simulink model "cdmatest3"  (R2020a)
settings: Solver=VariableStepAuto  StartTime=0.0  StopTime=10  RelTol=1e-3
libraries: commutil2 x20, commdigbbndpm3 x8, commrandsrc3 x8, commseqgen3 x8, commsink2 x4, dsparch4 x4, commchan3 x1
settings Model: Creator=xxy15334437753  LastModifiedBy=xxy15334437753

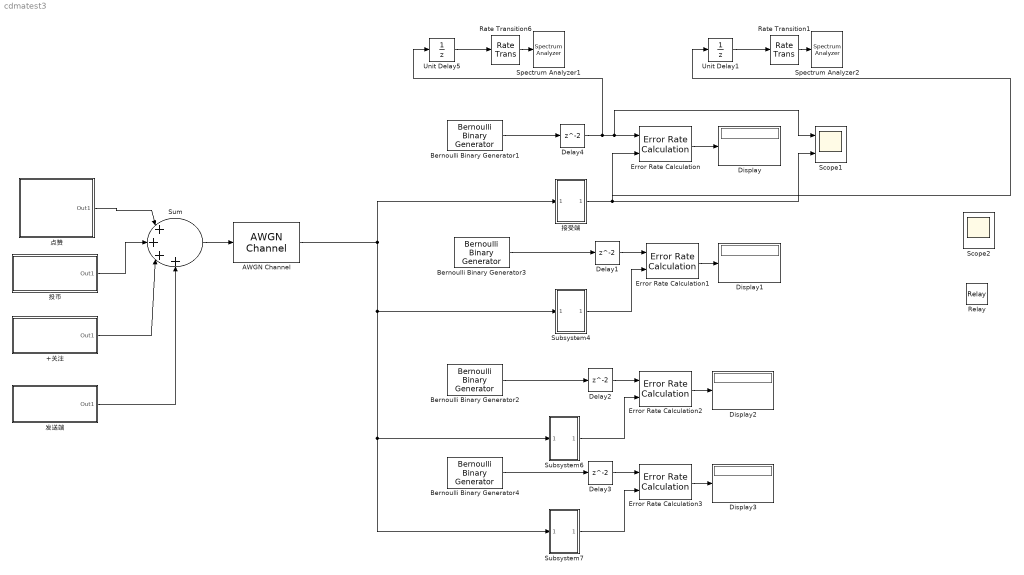
== system cdmatest3 ==
  +关注 : Subsystem
  AWGN Channel : commchan3/AWGN Channel  InputProcessing=Columns as channels (frame based)  seed=67  noiseMode="Signal to noise ratio  (Eb/No)"  EbNodB=10  EsNodB=10  SNRdB=20  bitsPerSym=1  Ps=1  Tsym=1/6400  variance=5
  Bernoulli Binary Generator1 : commrandsrc3/Bernoulli Binary Generator  ProbabilityOfZero=0.5  SeedSource=Parameter  Seed=88  SampleTime=0.01  SamplesPerFrame=1  OutputDataType=double  SimulateUsing=Code generation
  Bernoulli Binary Generator2 : commrandsrc3/Bernoulli Binary Generator  ProbabilityOfZero=0.5  SeedSource=Parameter  Seed=110  SampleTime=0.01  SamplesPerFrame=1  OutputDataType=double  SimulateUsing=Code generation
  Bernoulli Binary Generator3 : commrandsrc3/Bernoulli Binary Generator  ProbabilityOfZero=0.5  SeedSource=Parameter  Seed=67  SampleTime=0.01  SamplesPerFrame=1  OutputDataType=double  SimulateUsing=Code generation
  Bernoulli Binary Generator4 : commrandsrc3/Bernoulli Binary Generator  ProbabilityOfZero=0.5  SeedSource=Parameter  Seed=120  SampleTime=0.01  SamplesPerFrame=1  OutputDataType=double  SimulateUsing=Code generation
  Delay{1..4} (4 alike) : Delay
  Display{,1..3} (4 alike) : Display
  Error Rate Calculation{,1..3} (4 alike) : commsink2/Error Rate Calculation  N=0  st_delay=0  cp_mode=Entire frame  subframe=[]  PMode=Port  WsName=ErrorVec  RsMode2=off  stop=off  numErr=100  maxBits=1e6
  Rate Transition1 : RateTransition  OutPortSampleTime=1/3200
  Rate Transition6 : RateTransition  OutPortSampleTime=1/3200
  Relay : Relay
  Scope1 : Scope  NumInputPorts=2
  Scope2 : Scope  NumInputPorts=2
  Spectrum Analyzer1 : SpectrumAnalyzer
  Spectrum Analyzer2 : SpectrumAnalyzer
  Subsystem4 : Subsystem
  Subsystem6 : Subsystem
  Subsystem7 : Subsystem
  Sum : Sum  Inputs=|++++  OutMin=[-1]  OutMax=[1]  OutDataTypeStr=double
  Unit Delay1 : UnitDelay  SampleTime=-1  HasFrameUpgradeWarning=on
  Unit Delay5 : UnitDelay  SampleTime=-1  HasFrameUpgradeWarning=on
  发送端 : Subsystem
  投币 : Subsystem
  接受端 : Subsystem
  点赞 : Subsystem
  wires:
  Error Rate Calculation/1 -> Display/1
  Error Rate Calculation1/1 -> Display1/1
  Sum/1 -> AWGN Channel/1
  点赞/1(Out1) -> Sum/1
  投币/1(Out1) -> Sum/2
  +关注/1(Out1) -> Sum/3
  Bernoulli Binary Generator1/1 -> Delay4/1
  Bernoulli Binary Generator3/1 -> Delay1/1
  Delay1/1 -> Error Rate Calculation1/1
  Subsystem4/1(Out1) -> Error Rate Calculation1/2
  Subsystem6/1(Out1) -> Error Rate Calculation2/2
  Delay2/1 -> Error Rate Calculation2/1
  Bernoulli Binary Generator2/1 -> Delay2/1
  Error Rate Calculation2/1 -> Display2/1
  Error Rate Calculation3/1 -> Display3/1
  Bernoulli Binary Generator4/1 -> Delay3/1
  Delay3/1 -> Error Rate Calculation3/1
  Subsystem7/1(Out1) -> Error Rate Calculation3/2
  AWGN Channel/1 -> Subsystem7/1(In1), Subsystem6/1(In1), Subsystem4/1(In1), 接受端/1(In1)
  发送端/1(Out1) -> Sum/4
  Rate Transition6/1 -> Spectrum Analyzer1/1
  Delay4/1 -> Unit Delay5/1, Scope1/1, Error Rate Calculation/1
  Unit Delay5/1 -> Rate Transition6/1
  接受端/1(Out1) -> Unit Delay1/1, Scope1/2, Error Rate Calculation/2
  Rate Transition1/1 -> Spectrum Analyzer2/1
  Unit Delay1/1 -> Rate Transition1/1

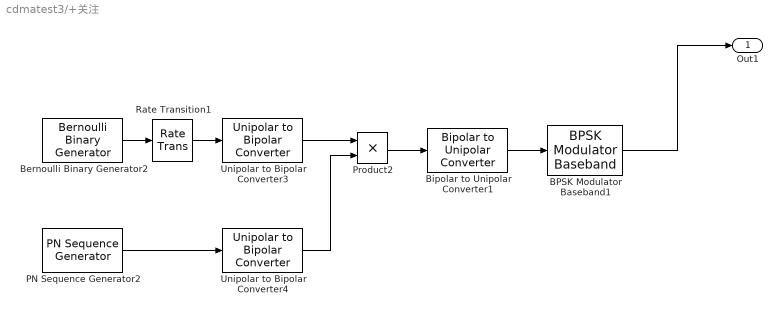
== system cdmatest3/+关注 ==
  BPSK Modulator Baseband1 : commdigbbndpm3/BPSK Modulator Baseband  Ph=0  outDtype=double  outWordLen=16  outUDDataType=sfix(16)  outFracLenMode=Best precision  outFracLen=15  outDataTypeStr=double  outLastDataTypeStr=double
  Bernoulli Binary Generator2 : commrandsrc3/Bernoulli Binary Generator  ProbabilityOfZero=0.5  SeedSource=Parameter  Seed=110  SampleTime=0.01  SamplesPerFrame=1  OutputDataType=double  SimulateUsing=Code generation
  Bipolar to Unipolar Converter1 : commutil2/Bipolar to Unipolar Converter  M=2  polarity=Positive  dataType=double
      settings: SourceProductBaseCode=CM
  PN Sequence Generator2 : commseqgen3/PN Sequence Generator  poly=[1 0 0 0 0 0 1 1]  ini_sta=[1 1 0 0 1 0 1]  outBitMaskSource=Dialog parameter  shift=0  outVarSiz=off  maxOutSizeMode=Dialog parameter  maxOutSize=[10 1]  Ts=1/6400  sampPerFrame=1  reset=off  bitPackedOutputs=off  outDataType=double  numPackedBits=8  bitPackDataSigned=off  bitPackedOutDType=double
  Product2 : Product
  Rate Transition1 : RateTransition  OutPortSampleTimeMultiple=20  OutPortSampleTime=1/3200
  Unipolar to Bipolar Converter3 : commutil2/Unipolar to Bipolar Converter  M=2  polarity=Positive  dataType=Inherit via internal rule
  Unipolar to Bipolar Converter4 : commutil2/Unipolar to Bipolar Converter  M=2  polarity=Positive  dataType=Inherit via internal rule
  Out1 : Outport
  wires:
  Rate Transition1/1 -> Unipolar to Bipolar Converter3/1
  BPSK Modulator Baseband1/1 -> Out1/1
  Bernoulli Binary Generator2/1 -> Rate Transition1/1
  Bipolar to Unipolar Converter1/1 -> BPSK Modulator Baseband1/1
  Unipolar to Bipolar Converter4/1 -> Product2/2
  Unipolar to Bipolar Converter3/1 -> Product2/1
  PN Sequence Generator2/1 -> Unipolar to Bipolar Converter4/1
  Product2/1 -> Bipolar to Unipolar Converter1/1

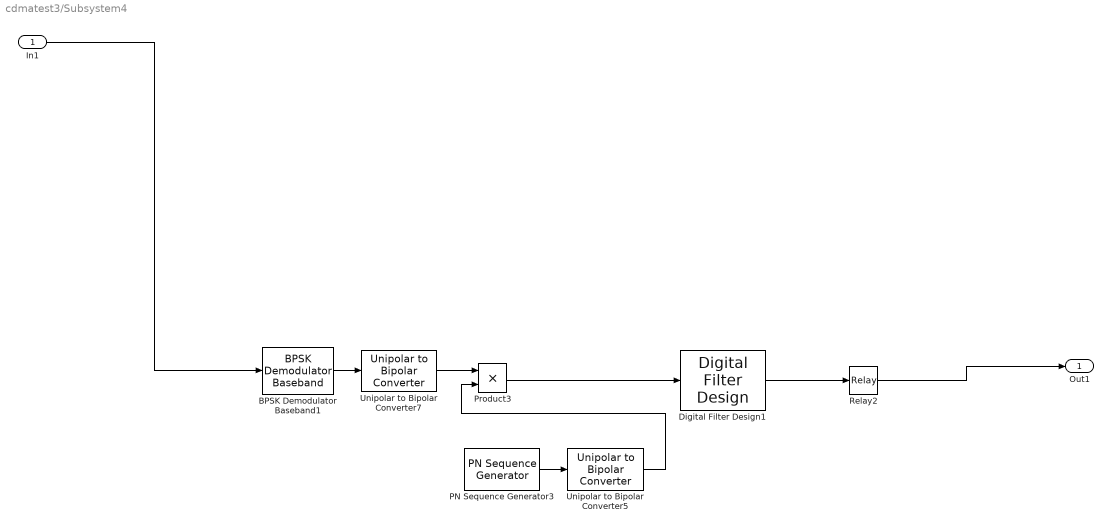
== system cdmatest3/Subsystem4 ==
  In1 : Inport
  BPSK Demodulator Baseband1 : commdigbbndpm3/BPSK Demodulator Baseband  DecType=Hard decision  VarSource=Dialog  Variance=1  Ph=0  outDtype=Inherit via internal rule  derotateFactorWordLen=16  derotateFactorDataTypeStr=Inherit: Same word length as input  derotateFactorLastDataTypeStr=Inherit: Same word length as input
  Digital Filter Design1 : dsparch4/Digital Filter Design  mwdsp_browser_bugfix_var=off
  PN Sequence Generator3 : commseqgen3/PN Sequence Generator  poly=[1 0 0 0 0 0 1 1]  ini_sta=[1 0 0 0 1 0 1]  outBitMaskSource=Dialog parameter  shift=0  outVarSiz=off  maxOutSizeMode=Dialog parameter  maxOutSize=[10 1]  Ts=1/6400  sampPerFrame=1  reset=off  bitPackedOutputs=off  outDataType=double  numPackedBits=8  bitPackDataSigned=off  bitPackedOutDType=double
  Product3 : Product
  Relay2 : Relay  OnSwitchValue=0  OffSwitchValue=0
  Unipolar to Bipolar Converter5 : commutil2/Unipolar to Bipolar Converter  M=2  polarity=Positive  dataType=Inherit via internal rule
  Unipolar to Bipolar Converter7 : commutil2/Unipolar to Bipolar Converter  M=2  polarity=Positive  dataType=Inherit via internal rule
  Out1 : Outport
  wires:
  PN Sequence Generator3/1 -> Unipolar to Bipolar Converter5/1
  In1/1 -> BPSK Demodulator Baseband1/1
  Product3/1 -> Digital Filter Design1/1
  Digital Filter Design1/1 -> Relay2/1
  Unipolar to Bipolar Converter5/1 -> Product3/2
  BPSK Demodulator Baseband1/1 -> Unipolar to Bipolar Converter7/1
  Unipolar to Bipolar Converter7/1 -> Product3/1
  Relay2/1 -> Out1/1

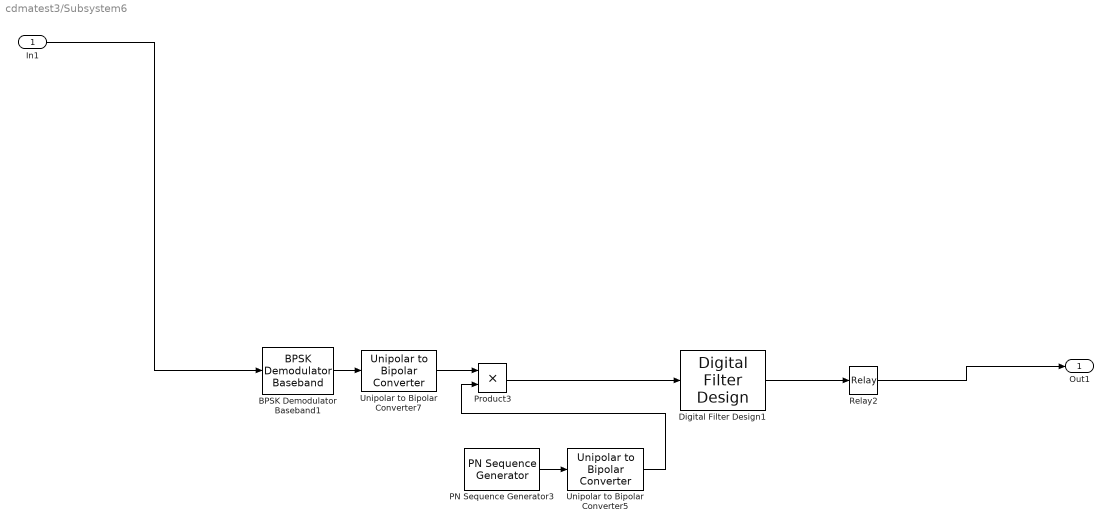
== system cdmatest3/Subsystem6 ==
  In1 : Inport
  BPSK Demodulator Baseband1 : commdigbbndpm3/BPSK Demodulator Baseband  DecType=Hard decision  VarSource=Dialog  Variance=1  Ph=0  outDtype=Inherit via internal rule  derotateFactorWordLen=16  derotateFactorDataTypeStr=Inherit: Same word length as input  derotateFactorLastDataTypeStr=Inherit: Same word length as input
  Digital Filter Design1 : dsparch4/Digital Filter Design  mwdsp_browser_bugfix_var=off
  PN Sequence Generator3 : commseqgen3/PN Sequence Generator  poly=[1 0 0 0 0 0 1 1]  ini_sta=[1 1 0 0 1 0 1]  outBitMaskSource=Dialog parameter  shift=0  outVarSiz=off  maxOutSizeMode=Dialog parameter  maxOutSize=[10 1]  Ts=1/6400  sampPerFrame=1  reset=off  bitPackedOutputs=off  outDataType=double  numPackedBits=8  bitPackDataSigned=off  bitPackedOutDType=double
  Product3 : Product
  Relay2 : Relay  OnSwitchValue=0  OffSwitchValue=0
  Unipolar to Bipolar Converter5 : commutil2/Unipolar to Bipolar Converter  M=2  polarity=Positive  dataType=Inherit via internal rule
  Unipolar to Bipolar Converter7 : commutil2/Unipolar to Bipolar Converter  M=2  polarity=Positive  dataType=Inherit via internal rule
  Out1 : Outport
  wires:
  Relay2/1 -> Out1/1
  Unipolar to Bipolar Converter7/1 -> Product3/1
  BPSK Demodulator Baseband1/1 -> Unipolar to Bipolar Converter7/1
  Unipolar to Bipolar Converter5/1 -> Product3/2
  Digital Filter Design1/1 -> Relay2/1
  Product3/1 -> Digital Filter Design1/1
  In1/1 -> BPSK Demodulator Baseband1/1
  PN Sequence Generator3/1 -> Unipolar to Bipolar Converter5/1

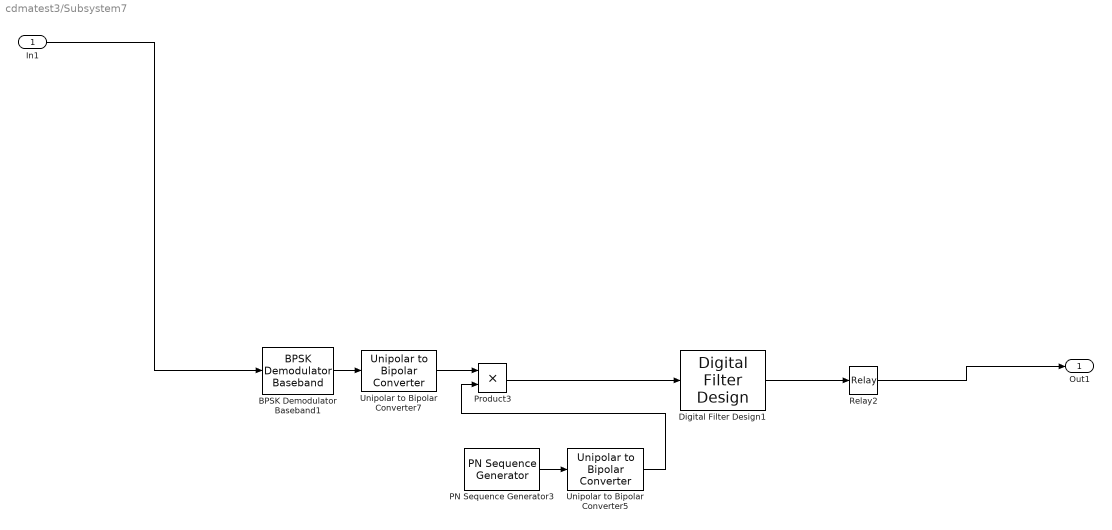
== system cdmatest3/Subsystem7 ==
  In1 : Inport
  BPSK Demodulator Baseband1 : commdigbbndpm3/BPSK Demodulator Baseband  DecType=Hard decision  VarSource=Dialog  Variance=1  Ph=0  outDtype=Inherit via internal rule  derotateFactorWordLen=16  derotateFactorDataTypeStr=Inherit: Same word length as input  derotateFactorLastDataTypeStr=Inherit: Same word length as input
  Digital Filter Design1 : dsparch4/Digital Filter Design  mwdsp_browser_bugfix_var=off
  PN Sequence Generator3 : commseqgen3/PN Sequence Generator  poly=[1 0 0 0 0 0 1 1]  ini_sta=[1 1 0 0 1 1 1]  outBitMaskSource=Dialog parameter  shift=0  outVarSiz=off  maxOutSizeMode=Dialog parameter  maxOutSize=[10 1]  Ts=1/6400  sampPerFrame=1  reset=off  bitPackedOutputs=off  outDataType=double  numPackedBits=8  bitPackDataSigned=off  bitPackedOutDType=double
  Product3 : Product
  Relay2 : Relay  OnSwitchValue=0  OffSwitchValue=0
  Unipolar to Bipolar Converter5 : commutil2/Unipolar to Bipolar Converter  M=2  polarity=Positive  dataType=Inherit via internal rule
  Unipolar to Bipolar Converter7 : commutil2/Unipolar to Bipolar Converter  M=2  polarity=Positive  dataType=Inherit via internal rule
  Out1 : Outport
  wires:
  PN Sequence Generator3/1 -> Unipolar to Bipolar Converter5/1
  In1/1 -> BPSK Demodulator Baseband1/1
  Product3/1 -> Digital Filter Design1/1
  Digital Filter Design1/1 -> Relay2/1
  Unipolar to Bipolar Converter5/1 -> Product3/2
  BPSK Demodulator Baseband1/1 -> Unipolar to Bipolar Converter7/1
  Unipolar to Bipolar Converter7/1 -> Product3/1
  Relay2/1 -> Out1/1

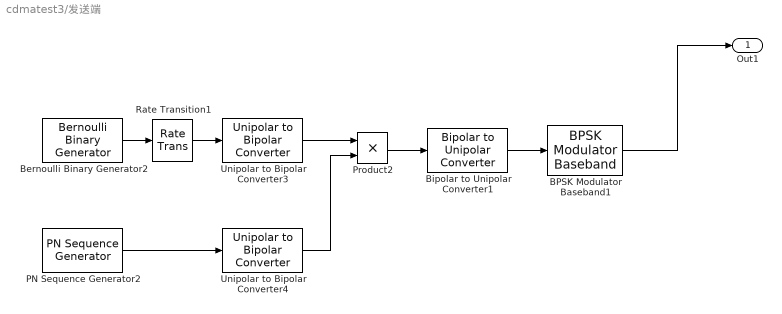
== system cdmatest3/发送端 ==
  BPSK Modulator Baseband1 : commdigbbndpm3/BPSK Modulator Baseband  Ph=0  outDtype=double  outWordLen=16  outUDDataType=sfix(16)  outFracLenMode=Best precision  outFracLen=15  outDataTypeStr=double  outLastDataTypeStr=double
  Bernoulli Binary Generator2 : commrandsrc3/Bernoulli Binary Generator  ProbabilityOfZero=0.5  SeedSource=Parameter  Seed=120  SampleTime=0.01  SamplesPerFrame=1  OutputDataType=double  SimulateUsing=Code generation
  Bipolar to Unipolar Converter1 : commutil2/Bipolar to Unipolar Converter  M=2  polarity=Positive  dataType=double
      settings: SourceProductBaseCode=CM
  PN Sequence Generator2 : commseqgen3/PN Sequence Generator  poly=[1 0 0 0 0 0 1 1]  ini_sta=[1 1 0 0 1 1 1]  outBitMaskSource=Dialog parameter  shift=0  outVarSiz=off  maxOutSizeMode=Dialog parameter  maxOutSize=[10 1]  Ts=1/6400  sampPerFrame=1  reset=off  bitPackedOutputs=off  outDataType=double  numPackedBits=8  bitPackDataSigned=off  bitPackedOutDType=double
  Product2 : Product
  Rate Transition1 : RateTransition  OutPortSampleTimeMultiple=20  OutPortSampleTime=1/3200
  Unipolar to Bipolar Converter3 : commutil2/Unipolar to Bipolar Converter  M=2  polarity=Positive  dataType=Inherit via internal rule
  Unipolar to Bipolar Converter4 : commutil2/Unipolar to Bipolar Converter  M=2  polarity=Positive  dataType=Inherit via internal rule
  Out1 : Outport
  wires:
  Product2/1 -> Bipolar to Unipolar Converter1/1
  PN Sequence Generator2/1 -> Unipolar to Bipolar Converter4/1
  Unipolar to Bipolar Converter3/1 -> Product2/1
  Unipolar to Bipolar Converter4/1 -> Product2/2
  Bipolar to Unipolar Converter1/1 -> BPSK Modulator Baseband1/1
  Bernoulli Binary Generator2/1 -> Rate Transition1/1
  BPSK Modulator Baseband1/1 -> Out1/1
  Rate Transition1/1 -> Unipolar to Bipolar Converter3/1

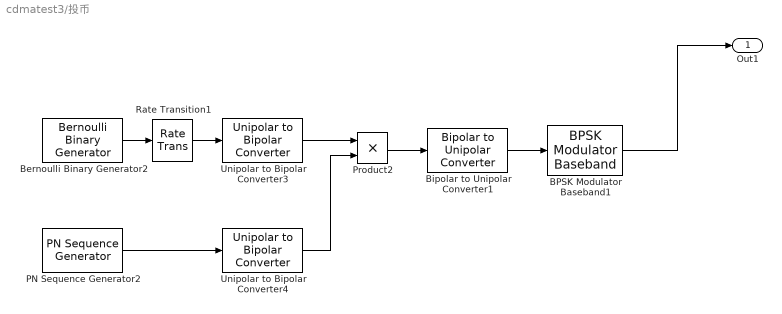
== system cdmatest3/投币 ==
  BPSK Modulator Baseband1 : commdigbbndpm3/BPSK Modulator Baseband  Ph=0  outDtype=double  outWordLen=16  outUDDataType=sfix(16)  outFracLenMode=Best precision  outFracLen=15  outDataTypeStr=double  outLastDataTypeStr=double
  Bernoulli Binary Generator2 : commrandsrc3/Bernoulli Binary Generator  ProbabilityOfZero=0.5  SeedSource=Parameter  Seed=67  SampleTime=0.01  SamplesPerFrame=1  OutputDataType=double  SimulateUsing=Code generation
  Bipolar to Unipolar Converter1 : commutil2/Bipolar to Unipolar Converter  M=2  polarity=Positive  dataType=double
      settings: SourceProductBaseCode=CM
  PN Sequence Generator2 : commseqgen3/PN Sequence Generator  poly=[1 0 0 0 0 0 1 1]  ini_sta=[1 0 0 0 1 0 1]  outBitMaskSource=Dialog parameter  shift=0  outVarSiz=off  maxOutSizeMode=Dialog parameter  maxOutSize=[10 1]  Ts=1/6400  sampPerFrame=1  reset=off  bitPackedOutputs=off  outDataType=double  numPackedBits=8  bitPackDataSigned=off  bitPackedOutDType=double
  Product2 : Product
  Rate Transition1 : RateTransition  OutPortSampleTimeMultiple=20  OutPortSampleTime=1/3200
  Unipolar to Bipolar Converter3 : commutil2/Unipolar to Bipolar Converter  M=2  polarity=Positive  dataType=Inherit via internal rule
  Unipolar to Bipolar Converter4 : commutil2/Unipolar to Bipolar Converter  M=2  polarity=Positive  dataType=Inherit via internal rule
  Out1 : Outport
  wires:
  Rate Transition1/1 -> Unipolar to Bipolar Converter3/1
  BPSK Modulator Baseband1/1 -> Out1/1
  Bernoulli Binary Generator2/1 -> Rate Transition1/1
  Bipolar to Unipolar Converter1/1 -> BPSK Modulator Baseband1/1
  Unipolar to Bipolar Converter4/1 -> Product2/2
  Unipolar to Bipolar Converter3/1 -> Product2/1
  PN Sequence Generator2/1 -> Unipolar to Bipolar Converter4/1
  Product2/1 -> Bipolar to Unipolar Converter1/1

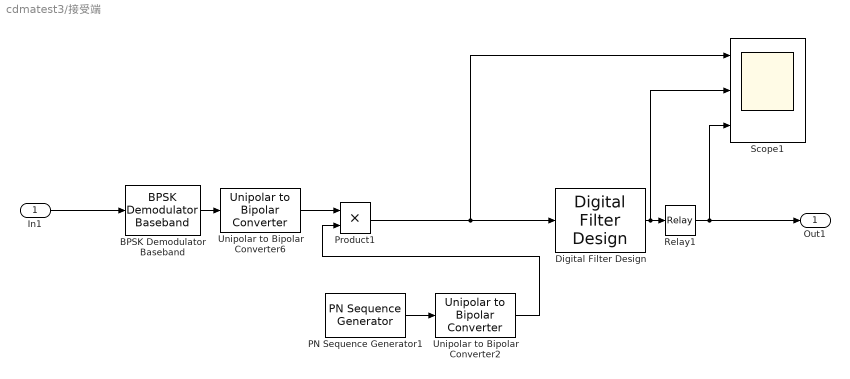
== system cdmatest3/接受端 ==
  In1 : Inport
  BPSK Demodulator Baseband : commdigbbndpm3/BPSK Demodulator Baseband  DecType=Hard decision  VarSource=Dialog  Variance=1  Ph=0  outDtype=Inherit via internal rule  derotateFactorWordLen=16  derotateFactorDataTypeStr=Inherit: Same word length as input  derotateFactorLastDataTypeStr=Inherit: Same word length as input
  Digital Filter Design : dsparch4/Digital Filter Design  mwdsp_browser_bugfix_var=off
  PN Sequence Generator1 : commseqgen3/PN Sequence Generator  poly=[1 0 0 0 0 0 1 1]  ini_sta=[1 0 0 0 0 0 0]  outBitMaskSource=Dialog parameter  shift=0  outVarSiz=off  maxOutSizeMode=Dialog parameter  maxOutSize=[10 1]  Ts=1/6400  sampPerFrame=1  reset=off  bitPackedOutputs=off  outDataType=double  numPackedBits=8  bitPackDataSigned=off  bitPackedOutDType=double
  Product1 : Product
  Relay1 : Relay  OnSwitchValue=0  OffSwitchValue=0
  Scope1 : Scope  NumInputPorts=3
  Unipolar to Bipolar Converter2 : commutil2/Unipolar to Bipolar Converter  M=2  polarity=Positive  dataType=Inherit via internal rule
  Unipolar to Bipolar Converter6 : commutil2/Unipolar to Bipolar Converter  M=2  polarity=Positive  dataType=Inherit via internal rule
  Out1 : Outport
  wires:
  Product1/1 -> Scope1/1, Digital Filter Design/1
  Relay1/1 -> Scope1/3, Out1/1
  Unipolar to Bipolar Converter6/1 -> Product1/1
  Digital Filter Design/1 -> Scope1/2, Relay1/1
  PN Sequence Generator1/1 -> Unipolar to Bipolar Converter2/1
  BPSK Demodulator Baseband/1 -> Unipolar to Bipolar Converter6/1
  Unipolar to Bipolar Converter2/1 -> Product1/2
  In1/1 -> BPSK Demodulator Baseband/1

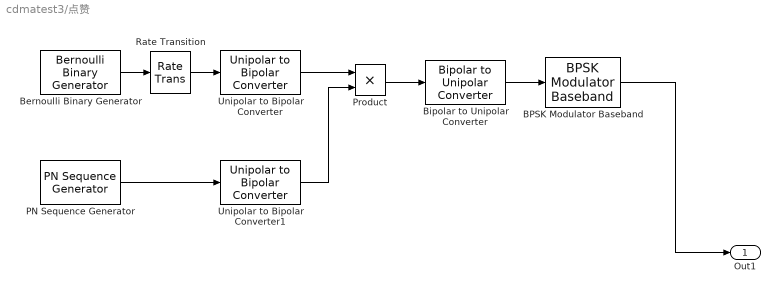
== system cdmatest3/点赞 ==
  BPSK Modulator Baseband : commdigbbndpm3/BPSK Modulator Baseband  Ph=0  outDtype=double  outWordLen=16  outUDDataType=sfix(16)  outFracLenMode=Best precision  outFracLen=15  outDataTypeStr=double  outLastDataTypeStr=double
  Bernoulli Binary Generator : commrandsrc3/Bernoulli Binary Generator  ProbabilityOfZero=0.5  SeedSource=Parameter  Seed=88  SampleTime=0.01  SamplesPerFrame=1  OutputDataType=double  SimulateUsing=Code generation
  Bipolar to Unipolar Converter : commutil2/Bipolar to Unipolar Converter  M=2  polarity=Positive  dataType=double
      settings: SourceProductBaseCode=CM
  PN Sequence Generator : commseqgen3/PN Sequence Generator  poly=[1 0 0 0 0 0 1 1]  ini_sta=[1 0 0 0 0 0 0]  outBitMaskSource=Dialog parameter  shift=0  outVarSiz=off  maxOutSizeMode=Dialog parameter  maxOutSize=[10 1]  Ts=1/6400  sampPerFrame=1  reset=off  bitPackedOutputs=off  outDataType=double  numPackedBits=8  bitPackDataSigned=off  bitPackedOutDType=double
  Product : Product
  Rate Transition : RateTransition  OutPortSampleTimeMultiple=20  OutPortSampleTime=1/6400
  Unipolar to Bipolar Converter : commutil2/Unipolar to Bipolar Converter  M=2  polarity=Positive  dataType=Inherit via internal rule
  Unipolar to Bipolar Converter1 : commutil2/Unipolar to Bipolar Converter  M=2  polarity=Positive  dataType=Inherit via internal rule
  Out1 : Outport
  wires:
  Rate Transition/1 -> Unipolar to Bipolar Converter/1
  Unipolar to Bipolar Converter1/1 -> Product/2
  PN Sequence Generator/1 -> Unipolar to Bipolar Converter1/1
  Product/1 -> Bipolar to Unipolar Converter/1
  Bernoulli Binary Generator/1 -> Rate Transition/1
  Unipolar to Bipolar Converter/1 -> Product/1
  BPSK Modulator Baseband/1 -> Out1/1
  Bipolar to Unipolar Converter/1 -> BPSK Modulator Baseband/1
